simulink model "TD4_Seance"  (Simulink 8.9)
settings: Solver=ode3  StartTime=0.0  StopTime=10  FixedStep=0.0001  RelTol=1e-3  EnableMultiTasking=on
settings Model: Creator=Eric  LastModifiedBy=telep
settings OptimizationCC: ExpressionDepthLimit=2147483647
settings DebuggingCC: SolverPrmCheckMsg=warning

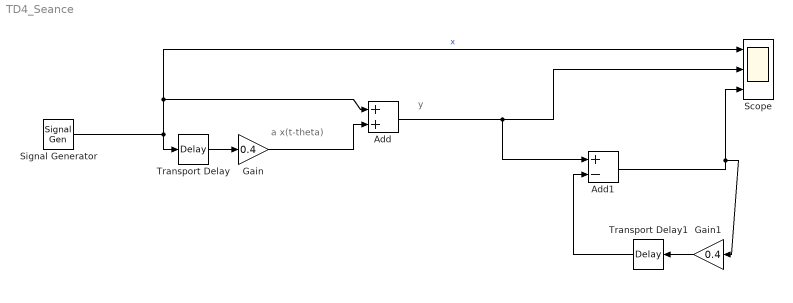
== system TD4_Seance ==
  note: y
  note: a x(t-theta)
  Add : Sum
  Add1 : Sum  Inputs=+-
  Gain : Gain  Gain=0.4
  Gain1 : Gain  Gain=0.4
  Scope : Scope  NumInputPorts=3
  Signal Generator : SignalGenerator  WaveForm=square  Frequency=2/3
  Transport Delay : TransportDelay  DelayTime=2
  Transport Delay1 : TransportDelay  DelayTime=2
  wires:
  Transport Delay/1 -> Gain/1
  Gain/1 -> Add/2
  Add/1 -> Add1/1, Scope/2
  Signal Generator/1 -> Transport Delay/1, Add/1, Scope/1  "x"
  Add1/1 -> Gain1/1, Scope/3
  Gain1/1 -> Transport Delay1/1
  Transport Delay1/1 -> Add1/2
